simulink model "eval_longitudinal_ctrl_pedalPos"  (R2019b)
settings: Solver=FixedStepDiscrete  StartTime=0.0  StopTime=inf  RelTol=1e-3  EnableMultiTasking=on
libraries: SCANeR_API x5
settings Model: Creator=sphilippe  LastModifiedBy=lpfeffer
settings DataIOCC: LimitDataPoints=on  SaveFormat=Array  ReturnWorkspaceOutputs=off
settings OptimizationCC: LifeSpan=inf
settings DebuggingCC: UnderspecifiedInitializationDetection=Classic  MergeDetectMultiDrivingBlocksExec=none  SolverPrmCheckMsg=warning  SFUnexpectedBacktrackingDiag=warning  SFNoUnconditionalDefaultTransitionDiag=warning  SFExecutionAtInitializationDiag=none  ArithmeticOperatorsInVariantConditions=warning
settings HardwareCC: ProdBitPerPointer=32  ProdBitPerSizeT=32  ProdBitPerPtrDiffT=32  ProdLargestAtomicFloat=None  ProdIntDivRoundTo=Undefined  ProdEndianess=Unspecified  ProdWordSize=32  ProdHWDeviceType=32-bit Generic
settings ModelReferenceCC: PropagateSignalLabelsOutOfModel=off
settings SFSimCC: SimUseLocalCustomCode=off  CustomCodeUndefinedFunction=UseInterfaceOnly
settings RTWCC: Description=SCANeR API Real-Time Target  SystemTargetFile=grt_scanerapi.tlc  TemplateMakefile=grt_scanerapi_vc.tmf  RTWUseLocalCustomCode=off
settings CodeAppCC: StateflowObjectComments=on
settings STFCustomTargetCC: GeneratePreprocessorConditionals=Disable all  MatFileLogging=on  CPPClassGenCompliant=on  GRTInterface=on  SystemTargetFile=grt_scanerapi.tlc
settings GRTTargetCC: TargetLangStandard=C89/C90 (ANSI)  ParMdlRefBuildCompliant=off  CompOptLevelCompliant=off  ConcurrentExecutionCompliant=off  GeneratePreprocessorConditionals=Disable all  CombineOutputUpdateFcns=off  GRTInterface=on  UseToolchainInfoCompliant=off
settings ConfigComp: CovMetricSettings=dw  CovHtmlReporting=on  CovSaveCumulativeToWorkspaceVar=on  CovSaveSingleToWorkspaceVar=on  CovExternalEMLEnable=off

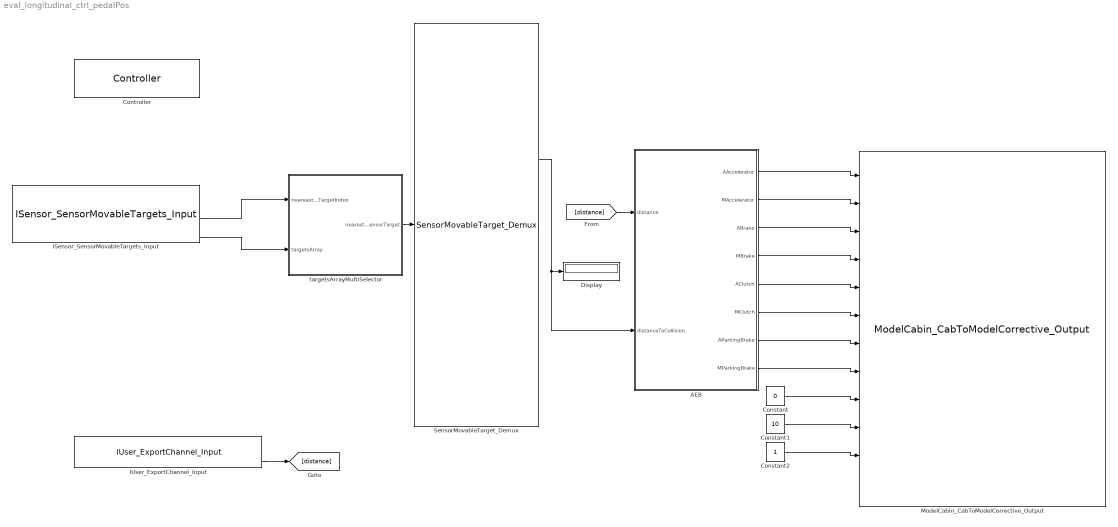
== system eval_longitudinal_ctrl_pedalPos ==
  AEB : MATLAB Function  TreatAsAtomicUnit=on
  Constant : Constant  Value=0
  Constant1 : Constant  Value=10
  Constant2 : Constant
  Controller : SCANeR_API/Controller  Priority=1  Config='SAMPLE_2022_ADAS'  ProcName='SIMULINK'  Frequency=100  NetworkOutputFrequency=10  TimeOut=30  IsSynchronized=off
      settings: SourceProductName=SCANeR API
  Display : Display
  ISensor_SensorMovableTargets_Input : SCANeR_API/Network inputs/ISensor/ISensor_SensorMovableTargets_Input  Priority=2  ev=off  globalId=300000
      settings: SourceProductName=SCANeR API
  IUser_ExportChannel_Input : SCANeR_API/Network inputs/IUser/IUser_ExportChannel_Input  Priority=2  ev=off  no=1000
      settings: SourceProductName=SCANeR API
  ModelCabin_CabToModelCorrective_Output : SCANeR_API/SHM outputs/ModelCabin/ModelCabin_CabToModelCorrective_Output  Priority=2  shmId=0
      settings: SourceProductName=SCANeR API
  SensorMovableTarget_Demux : SCANeR_API/Structures/SensorMovableTarget_Demux
      settings: SourceProductName=SCANeR API
  targetsArrayMultiSelector : Subsystem
  wires:
  ISensor_SensorMovableTargets_Input/6 -> targetsArrayMultiSelector/2(targetsArray)
  AEB/2(MAccelerator) -> ModelCabin_CabToModelCorrective_Output/2
  AEB/3(ABrake) -> ModelCabin_CabToModelCorrective_Output/3
  AEB/1(AAccelerator) -> ModelCabin_CabToModelCorrective_Output/1
  AEB/4(MBrake) -> ModelCabin_CabToModelCorrective_Output/4
  AEB/5(AClutch) -> ModelCabin_CabToModelCorrective_Output/5
  AEB/6(MClutch) -> ModelCabin_CabToModelCorrective_Output/6
  AEB/7(AParkingBrake) -> ModelCabin_CabToModelCorrective_Output/7
  AEB/8(MParkingBrake) -> ModelCabin_CabToModelCorrective_Output/8
  Constant/1 -> ModelCabin_CabToModelCorrective_Output/9
  Constant1/1 -> ModelCabin_CabToModelCorrective_Output/10
  Constant2/1 -> ModelCabin_CabToModelCorrective_Output/11
  [distance] -> AEB/1(distance)
  IUser_ExportChannel_Input/3 -> [distance]
  ISensor_SensorMovableTargets_Input/4 -> targetsArrayMultiSelector/1(neareastTargetIndex)
  targetsArrayMultiSelector/1(nearestSensorTarget) -> SensorMovableTarget_Demux/1
  SensorMovableTarget_Demux/15 -> Display/1, AEB/2(distanceToCollision)

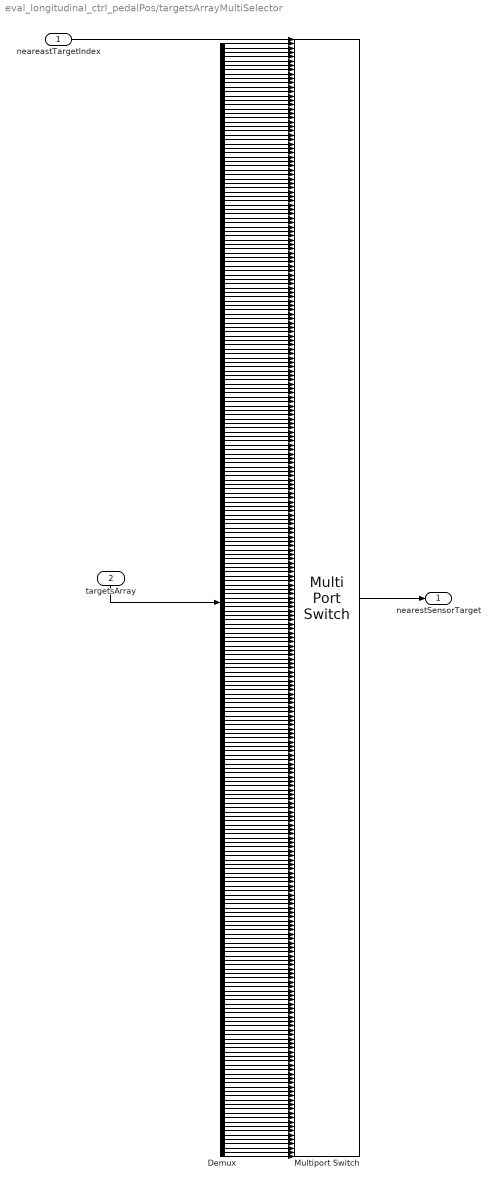
== system eval_longitudinal_ctrl_pedalPos/targetsArrayMultiSelector ==
  neareastTargetIndex : Inport
  targetsArray : Inport  Port=2
  Demux : Demux  Outputs=256
  Multiport Switch : MultiPortSwitch  DataPortOrder=Zero-based contiguous  Inputs=256  DiagnosticForDefault=None  zeroidx=on
  nearestSensorTarget : Outport
  wires:
  Demux/140 -> Multiport Switch/141
  Demux/137 -> Multiport Switch/138
  Demux/131 -> Multiport Switch/132
  Demux/90 -> Multiport Switch/91
  Demux/100 -> Multiport Switch/101
  Demux/110 -> Multiport Switch/111
  Demux/97 -> Multiport Switch/98
  Demux/116 -> Multiport Switch/117
  Demux/119 -> Multiport Switch/120
  Demux/91 -> Multiport Switch/92
  Demux/101 -> Multiport Switch/102
  Demux/117 -> Multiport Switch/118
  Demux/111 -> Multiport Switch/112
  Demux/112 -> Multiport Switch/113
  Demux/103 -> Multiport Switch/104
  Demux/109 -> Multiport Switch/110
  Demux/118 -> Multiport Switch/119
  Demux/115 -> Multiport Switch/116
  Demux/104 -> Multiport Switch/105
  Demux/98 -> Multiport Switch/99
  Demux/93 -> Multiport Switch/94
  Demux/95 -> Multiport Switch/96
  Demux/114 -> Multiport Switch/115
  Demux/113 -> Multiport Switch/114
  Demux/88 -> Multiport Switch/89
  Demux/133 -> Multiport Switch/134
  Demux/135 -> Multiport Switch/136
  Demux/159 -> Multiport Switch/160
  Demux/120 -> Multiport Switch/121
  Demux/143 -> Multiport Switch/144
  Demux/65 -> Multiport Switch/66
  Demux/59 -> Multiport Switch/60
  Demux/78 -> Multiport Switch/79
  Demux/32 -> Multiport Switch/33
  Demux/68 -> Multiport Switch/69
  Demux/29 -> Multiport Switch/30
  Demux/77 -> Multiport Switch/78
  Demux/76 -> Multiport Switch/77
  Demux/73 -> Multiport Switch/74
  Demux/61 -> Multiport Switch/62
  Demux/28 -> Multiport Switch/29
  Demux/69 -> Multiport Switch/70
  Demux/72 -> Multiport Switch/73
  Demux/75 -> Multiport Switch/76
  Demux/26 -> Multiport Switch/27
  Demux/38 -> Multiport Switch/39
  Demux/34 -> Multiport Switch/35
  Demux/23 -> Multiport Switch/24
  Demux/49 -> Multiport Switch/50
  Demux/41 -> Multiport Switch/42
  Demux/35 -> Multiport Switch/36
  Demux/45 -> Multiport Switch/46
  Demux/48 -> Multiport Switch/49
  Demux/40 -> Multiport Switch/41
  Demux/22 -> Multiport Switch/23
  Demux/30 -> Multiport Switch/31
  Demux/21 -> Multiport Switch/22
  Demux/31 -> Multiport Switch/32
  Demux/43 -> Multiport Switch/44
  Demux/24 -> Multiport Switch/25
  Demux/51 -> Multiport Switch/52
  Demux/27 -> Multiport Switch/28
  Demux/36 -> Multiport Switch/37
  Demux/52 -> Multiport Switch/53
  Demux/39 -> Multiport Switch/40
  Demux/37 -> Multiport Switch/38
  Demux/46 -> Multiport Switch/47
  Demux/42 -> Multiport Switch/43
  Demux/33 -> Multiport Switch/34
  Demux/50 -> Multiport Switch/51
  Demux/55 -> Multiport Switch/56
  Demux/47 -> Multiport Switch/48
  Demux/44 -> Multiport Switch/45
  Demux/25 -> Multiport Switch/26
  Demux/53 -> Multiport Switch/54
  Demux/54 -> Multiport Switch/55
  Demux/99 -> Multiport Switch/100
  Demux/105 -> Multiport Switch/106
  Demux/58 -> Multiport Switch/59
  Demux/56 -> Multiport Switch/57
  Demux/57 -> Multiport Switch/58
  Demux/81 -> Multiport Switch/82
  Demux/60 -> Multiport Switch/61
  Demux/64 -> Multiport Switch/65
  Demux/66 -> Multiport Switch/67
  Demux/67 -> Multiport Switch/68
  Demux/84 -> Multiport Switch/85
  Demux/71 -> Multiport Switch/72
  Demux/82 -> Multiport Switch/83
  Demux/83 -> Multiport Switch/84
  Demux/70 -> Multiport Switch/71
  Demux/63 -> Multiport Switch/64
  Demux/74 -> Multiport Switch/75
  Demux/79 -> Multiport Switch/80
  Demux/80 -> Multiport Switch/81
  Demux/62 -> Multiport Switch/63
  Demux/85 -> Multiport Switch/86
  Demux/86 -> Multiport Switch/87
  Demux/106 -> Multiport Switch/107
  Demux/107 -> Multiport Switch/108
  Demux/108 -> Multiport Switch/109
  targetsArray/1 -> Demux/1
  Multiport Switch/1 -> nearestSensorTarget/1
  neareastTargetIndex/1 -> Multiport Switch/1
  Demux/186 -> Multiport Switch/187
  Demux/182 -> Multiport Switch/183
  Demux/167 -> Multiport Switch/168
  Demux/141 -> Multiport Switch/142
  Demux/160 -> Multiport Switch/161
  Demux/172 -> Multiport Switch/173
  Demux/194 -> Multiport Switch/195
  Demux/185 -> Multiport Switch/186
  Demux/190 -> Multiport Switch/191
  Demux/188 -> Multiport Switch/189
  Demux/176 -> Multiport Switch/177
  Demux/162 -> Multiport Switch/163
  Demux/192 -> Multiport Switch/193
  Demux/163 -> Multiport Switch/164
  Demux/179 -> Multiport Switch/180
  Demux/168 -> Multiport Switch/169
  Demux/174 -> Multiport Switch/175
  Demux/191 -> Multiport Switch/192
  Demux/195 -> Multiport Switch/196
  Demux/150 -> Multiport Switch/151
  Demux/201 -> Multiport Switch/202
  Demux/193 -> Multiport Switch/194
  Demux/161 -> Multiport Switch/162
  Demux/202 -> Multiport Switch/203
  Demux/146 -> Multiport Switch/147
  Demux/165 -> Multiport Switch/166
  Demux/177 -> Multiport Switch/178
  Demux/181 -> Multiport Switch/182
  Demux/203 -> Multiport Switch/204
  Demux/204 -> Multiport Switch/205
  Demux/166 -> Multiport Switch/167
  Demux/180 -> Multiport Switch/181
  Demux/170 -> Multiport Switch/171
  Demux/206 -> Multiport Switch/207
  Demux/197 -> Multiport Switch/198
  Demux/208 -> Multiport Switch/209
  Demux/198 -> Multiport Switch/199
  Demux/219 -> Multiport Switch/220
  Demux/189 -> Multiport Switch/190
  Demux/226 -> Multiport Switch/227
  Demux/196 -> Multiport Switch/197
  Demux/200 -> Multiport Switch/201
  Demux/225 -> Multiport Switch/226
  Demux/171 -> Multiport Switch/172
  Demux/173 -> Multiport Switch/174
  Demux/250 -> Multiport Switch/251
  Demux/252 -> Multiport Switch/253
  Demux/213 -> Multiport Switch/214
  Demux/207 -> Multiport Switch/208
  Demux/175 -> Multiport Switch/176
  Demux/164 -> Multiport Switch/165
  Demux/212 -> Multiport Switch/213
  Demux/184 -> Multiport Switch/185
  Demux/223 -> Multiport Switch/224
  Demux/241 -> Multiport Switch/242
  Demux/234 -> Multiport Switch/235
  Demux/242 -> Multiport Switch/243
  Demux/178 -> Multiport Switch/179
  Demux/199 -> Multiport Switch/200
  Demux/169 -> Multiport Switch/170
  Demux/249 -> Multiport Switch/250
  Demux/187 -> Multiport Switch/188
  Demux/251 -> Multiport Switch/252
  Demux/183 -> Multiport Switch/184
  Demux/220 -> Multiport Switch/221
  Demux/218 -> Multiport Switch/219
  Demux/244 -> Multiport Switch/245
  Demux/230 -> Multiport Switch/231
  Demux/232 -> Multiport Switch/233
  Demux/243 -> Multiport Switch/244
  Demux/217 -> Multiport Switch/218
  Demux/216 -> Multiport Switch/217
  Demux/211 -> Multiport Switch/212
  Demux/214 -> Multiport Switch/215
  Demux/221 -> Multiport Switch/222
  Demux/248 -> Multiport Switch/249
  Demux/224 -> Multiport Switch/225
  Demux/236 -> Multiport Switch/237
  Demux/210 -> Multiport Switch/211
  Demux/229 -> Multiport Switch/230
  Demux/240 -> Multiport Switch/241
  Demux/215 -> Multiport Switch/216
  Demux/231 -> Multiport Switch/232
  Demux/237 -> Multiport Switch/238
  Demux/205 -> Multiport Switch/206
  Demux/239 -> Multiport Switch/240
  Demux/235 -> Multiport Switch/236
  Demux/245 -> Multiport Switch/246
  Demux/222 -> Multiport Switch/223
  Demux/227 -> Multiport Switch/228
  Demux/228 -> Multiport Switch/229
  Demux/209 -> Multiport Switch/210
  Demux/233 -> Multiport Switch/234
  Demux/238 -> Multiport Switch/239
  Demux/246 -> Multiport Switch/247
  Demux/247 -> Multiport Switch/248
  Demux/255 -> Multiport Switch/256
  Demux/10 -> Multiport Switch/11
  Demux/12 -> Multiport Switch/13
  Demux/16 -> Multiport Switch/17
  Demux/11 -> Multiport Switch/12
  Demux/6 -> Multiport Switch/7
  Demux/4 -> Multiport Switch/5
  Demux/19 -> Multiport Switch/20
  Demux/14 -> Multiport Switch/15
  Demux/253 -> Multiport Switch/254
  Demux/3 -> Multiport Switch/4
  Demux/5 -> Multiport Switch/6
  Demux/256 -> Multiport Switch/257
  Demux/7 -> Multiport Switch/8
  Demux/2 -> Multiport Switch/3
  Demux/8 -> Multiport Switch/9
  Demux/15 -> Multiport Switch/16
  Demux/1 -> Multiport Switch/2
  Demux/20 -> Multiport Switch/21
  Demux/254 -> Multiport Switch/255
  Demux/9 -> Multiport Switch/10
  Demux/13 -> Multiport Switch/14
  Demux/17 -> Multiport Switch/18
  Demux/18 -> Multiport Switch/19
  Demux/144 -> Multiport Switch/145
  Demux/153 -> Multiport Switch/154
  Demux/142 -> Multiport Switch/143
  Demux/138 -> Multiport Switch/139
  Demux/155 -> Multiport Switch/156
  Demux/128 -> Multiport Switch/129
  Demux/151 -> Multiport Switch/152
  Demux/149 -> Multiport Switch/150
  Demux/154 -> Multiport Switch/155
  Demux/148 -> Multiport Switch/149
  Demux/132 -> Multiport Switch/133
  Demux/145 -> Multiport Switch/146
  Demux/152 -> Multiport Switch/153
  Demux/147 -> Multiport Switch/148
  Demux/125 -> Multiport Switch/126
  Demux/94 -> Multiport Switch/95
  Demux/102 -> Multiport Switch/103
  Demux/96 -> Multiport Switch/97
  Demux/87 -> Multiport Switch/88
  Demux/89 -> Multiport Switch/90
  Demux/92 -> Multiport Switch/93
  Demux/122 -> Multiport Switch/123
  Demux/124 -> Multiport Switch/125
  Demux/126 -> Multiport Switch/127
  Demux/158 -> Multiport Switch/159
  Demux/129 -> Multiport Switch/130
  Demux/121 -> Multiport Switch/122
  Demux/134 -> Multiport Switch/135
  Demux/123 -> Multiport Switch/124
  Demux/156 -> Multiport Switch/157
  Demux/130 -> Multiport Switch/131
  Demux/136 -> Multiport Switch/137
  Demux/139 -> Multiport Switch/140
  Demux/157 -> Multiport Switch/158
  Demux/127 -> Multiport Switch/128

== matlab function eval_longitudinal_ctrl_pedalPos/AEB ==
  data: distance input; distanceToCollision input; AAccelerator output; MAccelerator output; ABrake output; MBrake output; AClutch output; MClutch output; AParkingBrake output; MParkingBrake output
function [AAccelerator, MAccelerator, ABrake, MBrake, AClutch, MClutch, AParkingBrake, MParkingBrake]= fcn(distance, distanceToCollision)
%#codegen
AAccelerator = 0;
MAccelerator = 1;
ABrake = 0;
MBrake = 1;
AClutch = 0;
MClutch = 1;
AParkingBrake = 0;
MParkingBrake = 1;

if(distanceToCollision ~= 0)
    if(distanceToCollision < distance)
        ABrake = 400;
    else
        ABrake = 0;
    end
end
